simulink model "Main"  (R2021b)
settings: Solver=VariableStepAuto  StartTime=0.0  StopTime=30  MaxStep=0.001  RelTol=1e-3
undefined symbols (not defined in the file): A, B, C, D, F, g, Ixx, Iyy, Izz, ka_lqr, ka_pp, kd_lqr, kd_pp, ks_lqr, ks_pp, L, Lf, m, Q1, Q2, T, u_EP, x_EP, y_EP
libraries: sim3dlib x1, uavsim3dlib x1, matrix_library x1, simulink x1
settings Model: Creator=sina.fazel  LastModifiedBy=Sepiamw

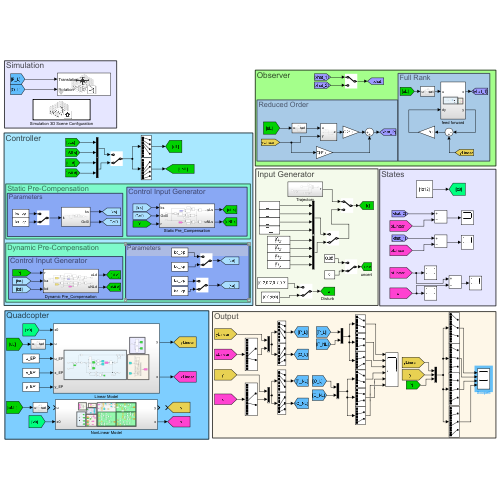
[thumbnail: Simulink's stored preview of the top-level diagram]
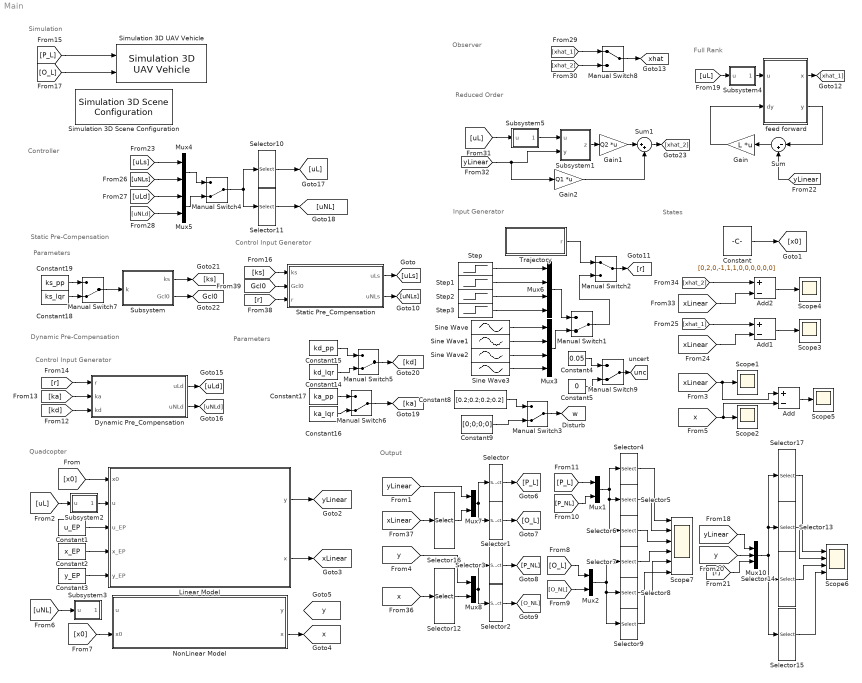
== system Main ==
  note: Full Rank
  note: Observer
  note: Simulation
  note: Control Input Generator
  note: Static Pre-Compensation
  note: Parameters
  note: Controller
  note: States
  note: Output
  note: Quadcopter
  note: Input Generator
  note: Control Input Generator
  note: Dynamic Pre-Compensation
  note: Parameters
  note: Reduced Order
  Add : Sum  Inputs=+-
  Add1 : Sum  Inputs=+-
  Add2 : Sum  Inputs=+-
  Constant : Constant  Value=[0,2,0,-1,1,1,0,0,0,0,0,0]
  Constant1 : Constant  Value=u_EP
  Constant14 : Constant  Value=kd_lqr  VectorParams1D=off
  Constant15 : Constant  Value=kd_pp  VectorParams1D=off
  Constant16 : Constant  Value=ka_lqr  VectorParams1D=off
  Constant17 : Constant  Value=ka_pp  VectorParams1D=off
  Constant18 : Constant  Value=ks_lqr
  Constant19 : Constant  Value=ks_pp
  Constant2 : Constant  Value=x_EP
  Constant3 : Constant  Value=y_EP
  Constant4 : Constant  Value=0.05
  Constant5 : Constant  Value=0
  Constant8 : Constant  Value=[0.2;0.2;0.2;0.2]
  Constant9 : Constant  Value=[0;0;0;0]
  Dynamic Pre_Compensation : Subsystem
  Gain : Gain  Gain=L  Multiplication=Matrix(K*u)
  Gain1 : Gain  Gain=Q2  Multiplication=Matrix(K*u)
  Gain2 : Gain  Gain=Q1  Multiplication=Matrix(K*u)
  Linear Model : Subsystem
  Manual Switch{1,3..7,9} (7 alike) : ManualSwitch  CurrentSetting=0
  Manual Switch2 : ManualSwitch
  Manual Switch8 : ManualSwitch
  Mux{1..2,4..5,7..8} (6 alike) : Mux  Inputs=2
  Mux10 : Mux  Inputs=3
  Mux3 : Mux
  Mux6 : Mux
  NonLinear Model : Subsystem
  Scope{1..5} (5 alike) : Scope
  Scope6 : Scope  NumInputPorts=4
  Scope7 : Scope  NumInputPorts=6
  Selector : Selector  InputPortWidth=6  IndexOptions=Index vector (dialog)  Indices=[1 2 3]  OutputSizes=1
  Selector1 : Selector  InputPortWidth=6  IndexOptions=Index vector (dialog)  Indices=[4 5 6]  OutputSizes=1
  Selector10 : Selector  InputPortWidth=8  IndexOptions=Index vector (dialog)  Indices=[1:4]  OutputSizes=1
  Selector11 : Selector  InputPortWidth=8  IndexOptions=Index vector (dialog)  Indices=[5:8]  OutputSizes=1
  Selector12 : Selector  InputPortWidth=12  IndexOptions=Index vector (dialog)  Indices=[7 8]  OutputSizes=1
  Selector13 : Selector  InputPortWidth=12  IndexOptions=Index vector (dialog)  Indices=[2,6,10]  OutputSizes=1
  Selector14 : Selector  InputPortWidth=12  IndexOptions=Index vector (dialog)  Indices=[3,7,11]  OutputSizes=1
  Selector15 : Selector  InputPortWidth=12  IndexOptions=Index vector (dialog)  Indices=[4,8,12]  OutputSizes=1
  Selector16 : Selector  InputPortWidth=12  IndexOptions=Index vector (dialog)  Indices=[7 8]  OutputSizes=1
  Selector17 : Selector  InputPortWidth=12  IndexOptions=Index vector (dialog)  Indices=[1,5,9]  OutputSizes=1
  Selector2 : Selector  InputPortWidth=6  IndexOptions=Index vector (dialog)  Indices=[4 5 6]  OutputSizes=1
  Selector3 : Selector  InputPortWidth=6  IndexOptions=Index vector (dialog)  Indices=[1 2 3]  OutputSizes=1
  Selector4 : Selector  InputPortWidth=6  IndexOptions=Index vector (dialog)  Indices=[1 4]  OutputSizes=1
  Selector5 : Selector  InputPortWidth=6  IndexOptions=Index vector (dialog)  Indices=[2 5]  OutputSizes=1
  Selector6 : Selector  InputPortWidth=6  IndexOptions=Index vector (dialog)  Indices=[3 6]  OutputSizes=1
  Selector7 : Selector  InputPortWidth=6  IndexOptions=Index vector (dialog)  Indices=[1 4]  OutputSizes=1
  Selector8 : Selector  InputPortWidth=6  IndexOptions=Index vector (dialog)  Indices=[2 5]  OutputSizes=1
  Selector9 : Selector  InputPortWidth=6  IndexOptions=Index vector (dialog)  Indices=[3 6]  OutputSizes=1
  Simulation 3D Scene Configuration : sim3dlib/Simulation 3D Scene Configuration  Priority=0  ProjectFormat_internal=Default Scenes  ProjectFormat=Default Scenes  SceneDesc=US city block  ProjectName=Q:\Matlab\toolbox\shared\sim3d_projects\automotive_project\UE4\WindowsNoEditor\VehicleSimulation.exe  ScenePath=/Game/Maps/USCityBlock  vehTagList={'Drone';'Scene Origin'}  vehTag=Drone  OpVisEn=off  Ts=1/60  EnableWindow=on  EnableWeather=off  SunAltitude=40.0  SunAzimuth=90  clouds=10  wind=1  fog=0  rain=0  sensorTag=MainCamera1  sensorId=1  sensorName=MainCamera1  mountLoc=Origin  offsetFlag=off  tmountOffset=[0, 0, 0]  rmountOffset=[0, 0, 0]  HorizontalResolution=1280  VerticalResolution=720  HorizontalFOV=60  mountPoint=[0 0 0]  mountOrientation=[0 0 0]  aMode=4  ID=1
      settings: SourceProductBaseCode=AE,DR,UV,VE
  Simulation 3D UAV Vehicle : uavsim3dlib/Simulation 3D UAV Vehicle  Priority=-1  Mesh=Quadrotor  MeshPath=/MathWorksUAVContent/UAVs/HexaRotorUAV/HexaRotor.HexaRotor  Color=Black  ActorName=Drone  InitialTranslation=[0 0 1]  InitialRotation=[0 0 0]  SampleTime=-1  ActorType=SimulinkVehicle  ID=C  aMode=4  ActorTag=Drone
      settings: SourceProductBaseCode=UV
  Sine Wave : Sin  Amplitude=0.5  Frequency=pi/8  Phase=pi/4  SampleTime=0
  Sine Wave1 : Sin  Amplitude=0.4  Frequency=pi/8  Phase=pi/8  SampleTime=0
  Sine Wave2 : Sin  Amplitude=1.5  Frequency=pi/8  SampleTime=0
  Sine Wave3 : Sin  Amplitude=0.02  Frequency=pi/16  Phase=pi/8  SampleTime=0
  Static Pre_Compensation : Subsystem
  Step : Step  Time=0  SampleTime=0
  Step1 : Step  Time=0  After=3  SampleTime=0
  Step2 : Step  Time=0  After=4  SampleTime=0
  Step3 : Step  Time=0  After=-pi/32  SampleTime=0
  Subsystem : Subsystem
  Subsystem1 : Subsystem
  Subsystem2 : Subsystem
  Subsystem3 : Subsystem
  Subsystem4 : Subsystem
  Subsystem5 : Subsystem
  Sum : Sum  Inputs=|-+
  Sum1 : Sum  Inputs=|++
  Trajectory : Subsystem
  feed forward : Subsystem
  tag scope: Gcl0=global, unc=global, w=global, x=global, xLinear=global, xhat=global, y=global, yLinear=global
  wires:
  Constant/1 -> [x0]
  Constant3/1 -> Linear Model/5(y_EP)
  Constant2/1 -> Linear Model/4(x_EP)
  Constant1/1 -> Linear Model/3(u_EP)
  Linear Model/1(y) -> [yLinear]
  Linear Model/2(x) -> [xLinear]
  [x0] -> Linear Model/1(x0)
  [xLinear] -> Add/1, Scope1/1
  [x] -> Add/2, Scope2/1
  Selector/1 -> [P_L]
  Selector1/1 -> [O_L]
  Selector3/1 -> [P_NL]
  Selector2/1 -> [O_NL]
  [P_NL] -> Mux1/2
  Add/1 -> Scope5/1
  [P_L] -> Mux1/1
  Mux1/1 -> Selector6/1, Selector5/1, Selector4/1
  Selector6/1 -> Scope7/3
  Selector5/1 -> Scope7/2
  Selector4/1 -> Scope7/1
  [O_L] -> Mux2/1
  [O_NL] -> Mux2/2
  Mux2/1 -> Selector7/1, Selector9/1, Selector8/1
  Selector7/1 -> Scope7/4
  Selector8/1 -> Scope7/5
  Selector9/1 -> Scope7/6
  Manual Switch1/1 -> Manual Switch2/2
  Mux3/1 -> Manual Switch1/2
  Sine Wave/1 -> Mux3/1
  Sine Wave1/1 -> Mux3/2
  Sine Wave2/1 -> Mux3/3
  [uNLs] -> Mux4/2
  [uLs] -> Mux4/1
  [uLd] -> Mux5/1
  [uNLd] -> Mux5/2
  Mux4/1 -> Manual Switch4/1
  Mux5/1 -> Manual Switch4/2
  Selector11/1 -> [uNL]
  Selector10/1 -> [uL]
  Manual Switch4/1 -> Selector10/1, Selector11/1
  Step3/1 -> Mux6/4
  Step2/1 -> Mux6/3
  Step1/1 -> Mux6/2
  Step/1 -> Mux6/1
  Mux6/1 -> Manual Switch1/1
  [y] -> Mux10/2
  [yLinear] -> Mux10/1
  Selector13/1 -> Scope6/2
  Selector15/1 -> Scope6/4
  Selector14/1 -> Scope6/3
  Mux10/1 -> Selector15/1, Selector14/1, Selector17/1, Selector13/1
  Constant8/1 -> Manual Switch3/1
  Constant9/1 -> Manual Switch3/2
  Manual Switch3/1 -> [w]
  Constant14/1 -> Manual Switch5/2
  Constant15/1 -> Manual Switch5/1
  Manual Switch5/1 -> [kd]
  Manual Switch6/1 -> [ka]
  Constant17/1 -> Manual Switch6/1
  Constant16/1 -> Manual Switch6/2
  Sine Wave3/1 -> Mux3/4
  Mux7/1 -> Selector1/1, Selector/1
  Mux8/1 -> Selector3/1, Selector2/1
  [y] -> Mux8/1
  [yLinear] -> Mux7/1
  [x] -> Selector12/1
  Selector12/1 -> Mux8/2
  [xLinear] -> Selector16/1
  Selector16/1 -> Mux7/2
  [r] -> Mux10/3
  Selector17/1 -> Scope6/1
  Constant18/1 -> Manual Switch7/2
  Constant19/1 -> Manual Switch7/1
  Manual Switch7/1 -> Subsystem/1(k)
  Subsystem/1(ks) -> [ks]
  Subsystem/2(Gcl0) -> [Gcl0]
  [ks] -> Static Pre_Compensation/1(ks)
  [r] -> Static Pre_Compensation/3(r)
  [Gcl0] -> Static Pre_Compensation/2(Gcl0)
  Static Pre_Compensation/1(uLs) -> [uLs]
  Static Pre_Compensation/2(uNLs) -> [uNLs]
  Dynamic Pre_Compensation/1(uLd) -> [uLd]
  Dynamic Pre_Compensation/2(uNLd) -> [uNLd]
  [kd] -> Dynamic Pre_Compensation/3(kd)
  [ka] -> Dynamic Pre_Compensation/2(ka)
  [r] -> Dynamic Pre_Compensation/1(r)
  Trajectory/1(r) -> Manual Switch2/1
  Manual Switch2/1 -> [r]
  [P_L] -> Simulation 3D UAV Vehicle/1
  [O_L] -> Simulation 3D UAV Vehicle/2
  NonLinear Model/2(x) -> [x]
  [x0] -> NonLinear Model/2(x0)
  feed forward/1(x) -> [xhat_1]
  feed forward/2(y) -> Sum/1
  [yLinear] -> Sum/2
  Sum/1 -> Gain/1
  Gain/1 -> feed forward/2(dy)
  [xhat_1] -> Add1/1
  [xLinear] -> Add1/2
  Add1/1 -> Scope3/1
  [xhat_1] -> Manual Switch8/1
  [xhat_2] -> Manual Switch8/2
  Manual Switch8/1 -> [xhat]
  [yLinear] -> Gain2/1, Subsystem1/2(y)
  Gain2/1 -> Sum1/2
  Subsystem1/1(z) -> Gain1/1
  Gain1/1 -> Sum1/1
  Sum1/1 -> [xhat_2]
  Add2/1 -> Scope4/1
  [xLinear] -> Add2/2
  [xhat_2] -> Add2/1
  Constant4/1 -> Manual Switch9/1
  Constant5/1 -> Manual Switch9/2
  Manual Switch9/1 -> [unc]
  Subsystem2/1(sat) -> Linear Model/2(u)
  [uL] -> Subsystem2/1(u)
  [uL] -> Subsystem4/1(u)
  Subsystem4/1(sat) -> feed forward/1(u)
  Subsystem5/1(sat) -> Subsystem1/1(u)
  [uL] -> Subsystem5/1(u)
  [uNL] -> Subsystem3/1(u)

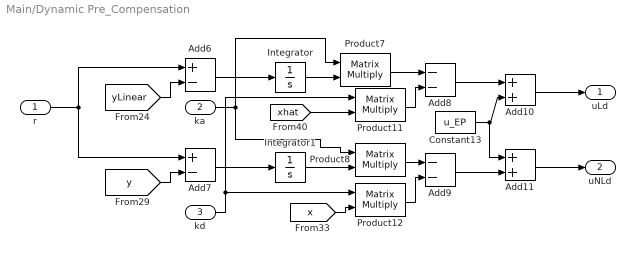
== system Main/Dynamic Pre_Compensation ==
  r : Inport
  ka : Inport  Port=2
  kd : Inport  Port=3
  Add10 : Sum
  Add11 : Sum
  Add6 : Sum  Inputs=+-
  Add7 : Sum  Inputs=+-
  Add8 : Sum  Inputs=--
  Add9 : Sum  Inputs=--
  Constant13 : Constant  Value=u_EP
  Integrator : Integrator
  Integrator1 : Integrator
  Product{7..8,11..12} (4 alike) : Product  Multiplication=Matrix(*)
  uLd : Outport
  uNLd : Outport  Port=2
  wires:
  Product12/1 -> Add9/2
  [xhat] -> Product11/2
  Product11/1 -> Add8/2
  kd/1 -> Product12/1, Product11/1
  ka/1 -> Product8/1, Product7/1
  [x] -> Product12/2
  Integrator/1 -> Product7/2
  Product7/1 -> Add8/1
  Constant13/1 -> Add11/1, Add10/2
  Add11/1 -> uNLd/1
  Add8/1 -> Add10/1
  Add9/1 -> Add11/2
  Integrator1/1 -> Product8/2
  Add10/1 -> uLd/1
  Product8/1 -> Add9/1
  Add7/1 -> Integrator1/1
  [y] -> Add7/2
  r/1 -> Add7/1, Add6/1
  [yLinear] -> Add6/2
  Add6/1 -> Integrator/1

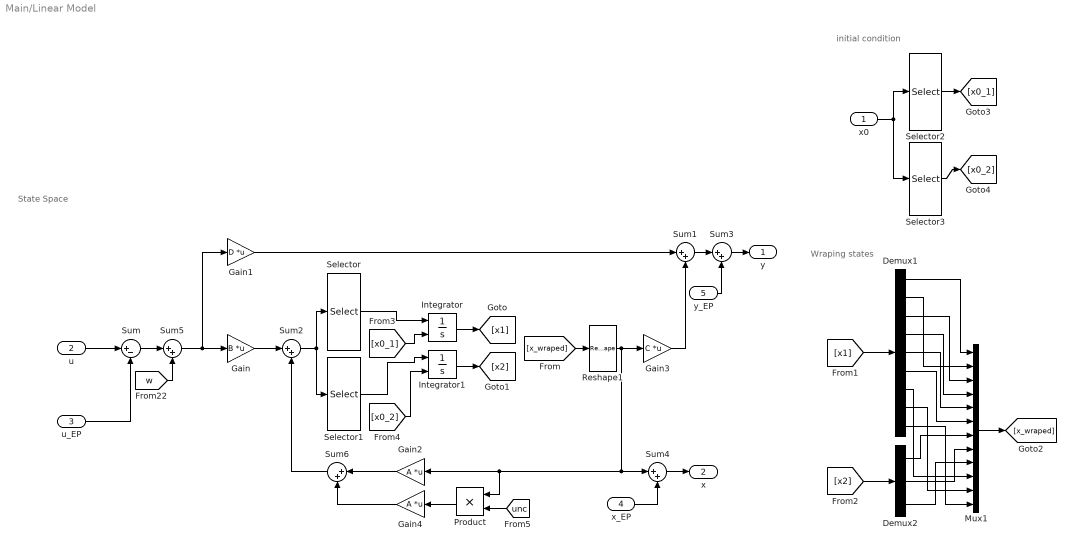
== system Main/Linear Model ==
  note: State Space
  note: Wraping states
  note: initial condition
  x0 : Inport
  u : Inport  Port=2
  u_EP : Inport  Port=3
  x_EP : Inport  Port=4
  y_EP : Inport  Port=5
  Demux1 : Demux  Outputs=9
  Demux2 : Demux  Outputs=3
  Gain : Gain  Gain=B  Multiplication=Matrix(K*u)
  Gain1 : Gain  Gain=D  Multiplication=Matrix(K*u)
  Gain2 : Gain  Gain=A  Multiplication=Matrix(K*u)
  Gain3 : Gain  Gain=C  Multiplication=Matrix(K*u)
  Gain4 : Gain  Gain=A  Multiplication=Matrix(K*u)
  Integrator : Integrator  InitialConditionSource=external
  Integrator1 : Integrator  InitialConditionSource=external  WrapState=on
  Mux1 : Mux  Inputs=12
  Product : Product
  Reshape1 : Reshape  OutputDimensionality=Column vector (2-D)
  Selector : Selector  InputPortWidth=12  IndexOptions=Index vector (dialog)  Indices=[1 2 3 4 5 6 10 11 12]  OutputSizes=1
  Selector1 : Selector  InputPortWidth=12  IndexOptions=Index vector (dialog)  Indices=[7 8 9]  OutputSizes=1
  Selector2 : Selector  InputPortWidth=12  IndexOptions=Index vector (dialog)  Indices=[1 2 3 4 5 6 10 11 12]  OutputSizes=1
  Selector3 : Selector  InputPortWidth=12  IndexOptions=Index vector (dialog)  Indices=[7 8 9]  OutputSizes=1
  Sum : Sum  Inputs=|+-
  Sum{1..6} (6 alike) : Sum  Inputs=|++
  y : Outport
  x : Outport  Port=2
  wires:
  [x1] -> Demux1/1
  Demux1/9 -> Mux1/12
  Demux1/5 -> Mux1/5
  [x2] -> Demux2/1
  Demux1/4 -> Mux1/4
  Demux2/2 -> Mux1/8
  Demux1/1 -> Mux1/1
  Demux1/7 -> Mux1/10
  Demux1/6 -> Mux1/6
  Demux1/3 -> Mux1/3
  Demux1/2 -> Mux1/2
  Demux2/3 -> Mux1/9
  Demux1/8 -> Mux1/11
  Demux2/1 -> Mux1/7
  Mux1/1 -> [x_wraped]
  x0/1 -> Selector3/1, Selector2/1
  Selector2/1 -> [x0_1]
  Selector3/1 -> [x0_2]
  Sum2/1 -> Selector1/1, Selector/1
  Selector/1 -> Integrator/1
  y_EP/1 -> Sum3/2
  Gain1/1 -> Sum1/1
  Sum3/1 -> y/1
  Gain/1 -> Sum2/1
  x_EP/1 -> Sum4/2
  Selector1/1 -> Integrator1/1
  [x0_1] -> Integrator/2
  [x0_2] -> Integrator1/2
  u/1 -> Sum/1
  Integrator/1 -> [x1]
  Sum1/1 -> Sum3/1
  Integrator1/1 -> [x2]
  u_EP/1 -> Sum/2
  Gain3/1 -> Sum1/2
  Sum4/1 -> x/1
  Sum/1 -> Sum5/1
  Sum5/1 -> Gain1/1, Gain/1
  [x_wraped] -> Reshape1/1
  Reshape1/1 -> Sum4/1, Product/1, Gain2/1, Gain3/1
  [w] -> Sum5/2
  Gain2/1 -> Sum6/1
  Sum6/1 -> Sum2/2
  Product/1 -> Gain4/1
  Gain4/1 -> Sum6/2
  [unc] -> Product/2

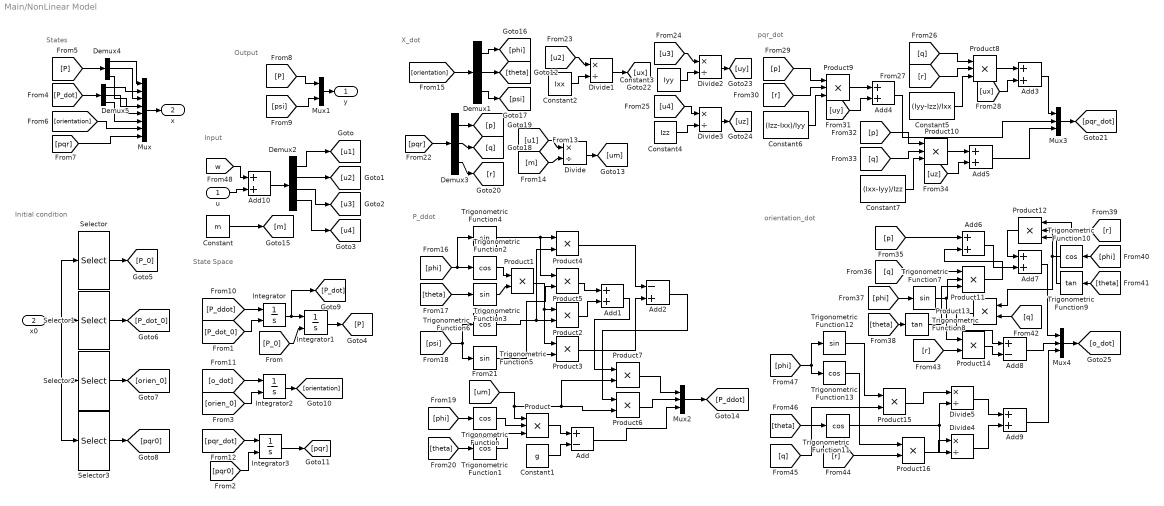
== system Main/NonLinear Model ==
  note: X_dot
  note: P_ddot
  note: State Space
  note: Output
  note: States
  note: Input
  note: Initial condition
  note: pqr_dot
  note: orientation_dot
  u : Inport
  x0 : Inport  Port=2
  Add : Sum  Inputs=+-
  Add{1,3..7,9..10} (8 alike) : Sum
  Add2 : Sum  Inputs=-+
  Add8 : Sum  Inputs=+-
  Constant : Constant  Value=m
  Constant1 : Constant  Value=g
  Constant2 : Constant  Value=Ixx
  Constant3 : Constant  Value=Iyy
  Constant4 : Constant  Value=Izz
  Constant5 : Constant  Value=(Iyy-Izz)/Ixx
  Constant6 : Constant  Value=(Izz-Ixx)/Iyy
  Constant7 : Constant  Value=(Ixx-Iyy)/Izz
  Demux{1,3..5} (4 alike) : Demux  Outputs=3
  Demux2 : Demux
  Divide{,1..5} (6 alike) : Product  Inputs=*/
  Integrator : Integrator  InitialConditionSource=external
  Integrator1 : Integrator  InitialConditionSource=external
  Integrator2 : Integrator  InitialConditionSource=external  WrapState=on
  Integrator3 : Integrator  InitialConditionSource=external
  Mux : Mux  Inputs=8
  Mux1 : Mux  Inputs=2
  Mux2 : Mux  Inputs=3
  Mux3 : Mux  Inputs=3
  Mux4 : Mux  Inputs=3
  Product{,8..12} (6 alike) : Product  Inputs=3
  Product{1..7,13..16} (11 alike) : Product
  Selector : Selector  InputPortWidth=12  IndexOptions=Index vector (dialog)  Indices=[1 3 5]  OutputSizes=1
  Selector1 : Selector  InputPortWidth=12  IndexOptions=Index vector (dialog)  Indices=[2 4 6]  OutputSizes=1
  Selector2 : Selector  InputPortWidth=12  IndexOptions=Index vector (dialog)  Indices=[7 8 9]  OutputSizes=1
  Selector3 : Selector  InputPortWidth=12  IndexOptions=Index vector (dialog)  Indices=[10 11 12]  OutputSizes=1
  Trigonometric Function{,1..2,6,10..11,13} (7 alike) : Trigonometry  Operator=cos
  Trigonometric Function{3..5,7,12} (5 alike) : Trigonometry
  Trigonometric Function8 : Trigonometry  Operator=tan
  Trigonometric Function9 : Trigonometry  Operator=tan
  y : Outport
  x : Outport  Port=2
  wires:
  x0/1 -> Selector3/1, Selector2/1, Selector1/1, Selector/1
  u/1 -> Add10/2
  Demux2/1 -> [u1]
  Demux2/4 -> [u4]
  Demux2/3 -> [u3]
  Demux2/2 -> [u2]
  Integrator/1 -> [P_dot], Integrator1/1
  Selector/1 -> [P_0]
  Selector1/1 -> [P_dot_0]
  [P_0] -> Integrator1/2
  [P_dot_0] -> Integrator/2
  Selector2/1 -> [orien_0]
  Selector3/1 -> [pqr0]
  [pqr0] -> Integrator3/2
  [orien_0] -> Integrator2/2
  Integrator1/1 -> [P]
  Integrator2/1 -> [orientation]
  Integrator3/1 -> [pqr]
  [pqr] -> Mux/8
  [orientation] -> Mux/7
  [P_dot] -> Demux5/1
  [P] -> Demux4/1
  Mux/1 -> x/1
  Mux1/1 -> y/1
  [P] -> Mux1/1
  [P_ddot] -> Integrator/1
  [o_dot] -> Integrator2/1
  [pqr_dot] -> Integrator3/1
  Constant/1 -> [m]
  [u1] -> Divide/1
  Demux1/3 -> [psi]
  Demux1/2 -> [theta]
  Demux1/1 -> [phi]
  [m] -> Divide/2
  Divide/1 -> [um]
  [orientation] -> Demux1/1
  [phi] -> Trigonometric Function/1
  [theta] -> Trigonometric Function1/1
  [um] -> Product7/2, Product6/2, Product/1
  Trigonometric Function/1 -> Product/2
  Trigonometric Function1/1 -> Product/3
  Product/1 -> Add/1
  Constant1/1 -> Add/2
  [pqr] -> Demux3/1
  Demux3/2 -> [q]
  Demux3/3 -> [r]
  Demux3/1 -> [p]
  Add/1 -> Mux2/3
  Mux2/1 -> [P_ddot]
  [phi] -> Trigonometric Function4/1, Trigonometric Function2/1
  [theta] -> Trigonometric Function3/1
  Trigonometric Function2/1 -> Product1/1
  Trigonometric Function3/1 -> Product1/2
  [psi] -> Trigonometric Function5/1, Trigonometric Function6/1
  Product1/1 -> Product3/1, Product2/1
  Trigonometric Function6/1 -> Product4/2, Product2/2
  Trigonometric Function5/1 -> Product3/2, Product5/2
  Trigonometric Function4/1 -> Product5/1, Product4/1
  Product2/1 -> Add1/2
  Product5/1 -> Add1/1
  Product3/1 -> Add2/2
  Product4/1 -> Add2/1
  Product7/1 -> Mux2/1
  Product6/1 -> Mux2/2
  Add2/1 -> Product6/1
  Add1/1 -> Product7/1
  Mux3/1 -> [pqr_dot]
  Constant4/1 -> Divide3/2
  Constant3/1 -> Divide2/2
  [u4] -> Divide3/1
  [u3] -> Divide2/1
  [u2] -> Divide1/1
  Constant2/1 -> Divide1/2
  Divide1/1 -> [ux]
  Divide2/1 -> [uy]
  Divide3/1 -> [uz]
  [q] -> Product8/1
  [r] -> Product8/2
  Product8/1 -> Add3/1
  Constant5/1 -> Product8/3
  [ux] -> Add3/2
  Add3/1 -> Mux3/1
  [uy] -> Add4/2
  Constant6/1 -> Product9/3
  Product9/1 -> Add4/1
  [r] -> Product9/2
  [p] -> Product9/1
  Add4/1 -> Mux3/2
  [p] -> Product10/1
  [q] -> Product10/2
  Product10/1 -> Add5/1
  Constant7/1 -> Product10/3
  [uz] -> Add5/2
  Add5/1 -> Mux3/3
  Mux4/1 -> [o_dot]
  [p] -> Add6/1
  [q] -> Product11/1
  Product11/1 -> Add6/2
  Trigonometric Function7/1 -> Product14/1, Product11/2
  [phi] -> Trigonometric Function7/1
  [theta] -> Trigonometric Function8/1
  Trigonometric Function8/1 -> Product11/3
  Add6/1 -> Add7/2
  Add7/1 -> Mux4/1
  [theta] -> Trigonometric Function9/1
  Product12/1 -> Add7/1
  [phi] -> Trigonometric Function10/1
  Trigonometric Function10/1 -> Product13/1, Product12/2
  Trigonometric Function9/1 -> Product12/3
  [r] -> Product12/1
  [q] -> Product13/2
  Add8/1 -> Mux4/2
  Product13/1 -> Add8/1
  Product14/1 -> Add8/2
  [r] -> Product14/2
  Add9/1 -> Mux4/3
  [r] -> Product16/2
  [q] -> Product15/2
  [theta] -> Trigonometric Function11/1
  Trigonometric Function11/1 -> Divide4/2, Divide5/2
  Product16/1 -> Divide4/1
  Product15/1 -> Divide5/1
  Divide5/1 -> Add9/1
  Divide4/1 -> Add9/2
  [phi] -> Trigonometric Function12/1, Trigonometric Function13/1
  Trigonometric Function12/1 -> Product15/1
  Trigonometric Function13/1 -> Product16/1
  Demux5/3 -> Mux/6
  Demux5/2 -> Mux/4
  Demux5/1 -> Mux/2
  Demux4/1 -> Mux/1
  Demux4/2 -> Mux/3
  Demux4/3 -> Mux/5
  Add10/1 -> Demux2/1
  [w] -> Add10/1
  [psi] -> Mux1/2

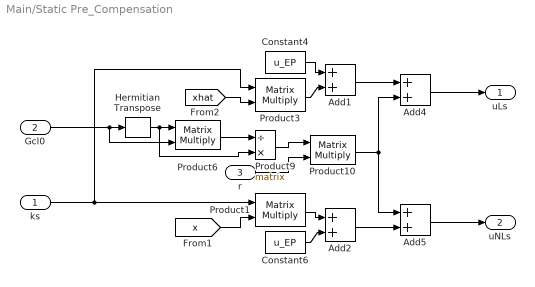
== system Main/Static Pre_Compensation ==
  ks : Inport
  Gcl0 : Inport  Port=2
  r : Inport  Port=3
  Add{1..2,4..5} (4 alike) : Sum
  Constant4 : Constant  Value=u_EP
  Constant6 : Constant  Value=u_EP
  Hermitian Transpose : matrix_library/Hermitian Transpose
      settings: SourceProductBaseCode=SL
  Product{1,3,6,10} (4 alike) : Product  Multiplication=Matrix(*)
  Product9 : Product  Inputs=/*  Multiplication=Matrix(*)
  uLs : Outport
  uNLs : Outport  Port=2
  wires:
  Gcl0/1 -> Product6/2, Hermitian Transpose/1
  Product6/1 -> Product9/1
  [xhat] -> Product3/2
  ks/1 -> Product1/1, Product3/1
  Product1/1 -> Add2/1
  Product9/1 -> Product10/1
  Constant4/1 -> Add1/1
  r/1 -> Product10/2
  [x] -> Product1/2
  Hermitian Transpose/1 -> Product9/2, Product6/1
  Add2/1 -> Add5/2
  Add1/1 -> Add4/1
  Add5/1 -> uNLs/1
  Product10/1 -> Add4/2, Add5/1
  Product3/1 -> Add1/2
  Add4/1 -> uLs/1
  Constant6/1 -> Add2/2

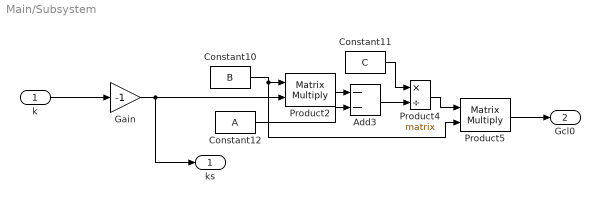
== system Main/Subsystem ==
  k : Inport
  Add3 : Sum  Inputs=--
  Constant10 : Constant  Value=B  VectorParams1D=off
  Constant11 : Constant  Value=C  VectorParams1D=off
  Constant12 : Constant  Value=A  VectorParams1D=off
  Gain : Gain  Gain=-1
  Product2 : Product  Multiplication=Matrix(*)
  Product4 : Product  Inputs=*/  Multiplication=Matrix(*)
  Product5 : Product  Multiplication=Matrix(*)
  ks : Outport
  Gcl0 : Outport  Port=2
  wires:
  Constant10/1 -> Product2/1, Product5/2
  Add3/1 -> Product4/2
  Gain/1 -> ks/1, Product2/2
  Constant11/1 -> Product4/1
  Product2/1 -> Add3/1
  Constant12/1 -> Add3/2
  Product5/1 -> Gcl0/1
  Product4/1 -> Product5/1
  k/1 -> Gain/1

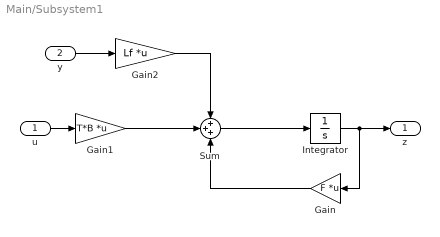
== system Main/Subsystem1 ==
  u : Inport
  y : Inport  Port=2
  Gain : Gain  Gain=F  Multiplication=Matrix(K*u)
  Gain1 : Gain  Gain=T*B  Multiplication=Matrix(K*u)
  Gain2 : Gain  Gain=Lf  Multiplication=Matrix(K*u)
  Integrator : Integrator
  Sum : Sum  Inputs=+++
  z : Outport
  wires:
  Integrator/1 -> Gain/1, z/1
  Sum/1 -> Integrator/1
  Gain/1 -> Sum/3
  Gain1/1 -> Sum/2
  u/1 -> Gain1/1
  y/1 -> Gain2/1
  Gain2/1 -> Sum/1

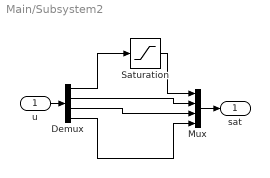
== system Main/Subsystem2 ==
  u : Inport
  Demux : Demux
  Mux : Mux
  Saturation : Saturate  UpperLimit=35  LowerLimit=0
  sat : Outport
  wires:
  Demux/4 -> Mux/4
  Demux/3 -> Mux/3
  Demux/2 -> Mux/2
  Saturation/1 -> Mux/1
  Demux/1 -> Saturation/1
  u/1 -> Demux/1
  Mux/1 -> sat/1

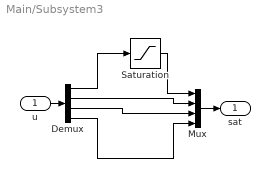
== system Main/Subsystem3 ==
  u : Inport
  Demux : Demux
  Mux : Mux
  Saturation : Saturate  UpperLimit=25  LowerLimit=0
  sat : Outport
  wires:
  Demux/4 -> Mux/4
  Demux/3 -> Mux/3
  Demux/2 -> Mux/2
  Saturation/1 -> Mux/1
  Demux/1 -> Saturation/1
  u/1 -> Demux/1
  Mux/1 -> sat/1

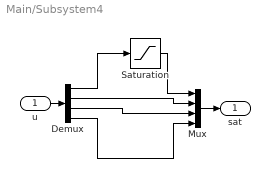
== system Main/Subsystem4 ==
  u : Inport
  Demux : Demux
  Mux : Mux
  Saturation : Saturate  UpperLimit=35  LowerLimit=0
  sat : Outport
  wires:
  Demux/4 -> Mux/4
  Demux/3 -> Mux/3
  Demux/2 -> Mux/2
  Saturation/1 -> Mux/1
  Demux/1 -> Saturation/1
  u/1 -> Demux/1
  Mux/1 -> sat/1

== system Main/Subsystem5 ==
  u : Inport
  Demux : Demux
  Mux : Mux
  Saturation : Saturate  UpperLimit=25  LowerLimit=0
  sat : Outport
  wires:
  Demux/4 -> Mux/4
  Demux/3 -> Mux/3
  Demux/2 -> Mux/2
  Saturation/1 -> Mux/1
  Demux/1 -> Saturation/1
  u/1 -> Demux/1
  Mux/1 -> sat/1

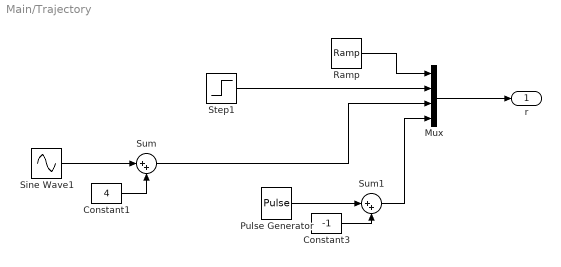
== system Main/Trajectory ==
  Constant1 : Constant  Value=4
  Constant3 : Constant  Value=-1
  Mux : Mux
  Pulse Generator : DiscretePulseGenerator  PulseType=Time based  Amplitude=2  Period=8  PulseWidth=50
  Ramp : simulink/Sources/Ramp  slope=4  start=0  InitialOutput=0
  Sine Wave1 : Sin  Amplitude=2  Frequency=pi/4  SampleTime=0
  Step1 : Step  Time=4  SampleTime=0
  Sum : Sum  Inputs=|++
  Sum1 : Sum  Inputs=|++
  r : Outport
  wires:
  Mux/1 -> r/1
  Sum1/1 -> Mux/4
  Sine Wave1/1 -> Sum/1
  Constant1/1 -> Sum/2
  Constant3/1 -> Sum1/2
  Pulse Generator/1 -> Sum1/1
  Sum/1 -> Mux/3
  Step1/1 -> Mux/2
  Ramp/1 -> Mux/1

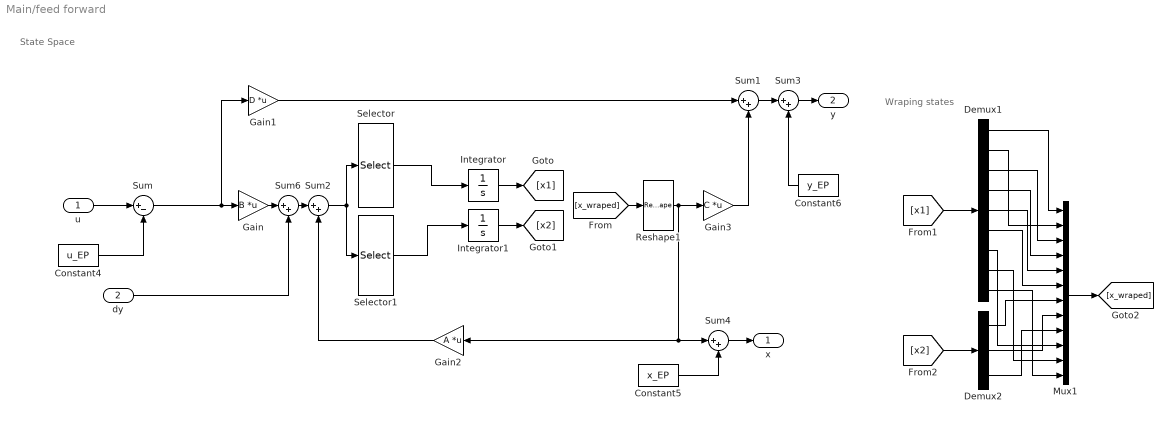
== system Main/feed forward ==
  note: Wraping states
  note: State Space
  u : Inport
  dy : Inport  Port=2
  Constant4 : Constant  Value=u_EP
  Constant5 : Constant  Value=x_EP
  Constant6 : Constant  Value=y_EP
  Demux1 : Demux  Outputs=9
  Demux2 : Demux  Outputs=3
  Gain : Gain  Gain=B  Multiplication=Matrix(K*u)
  Gain1 : Gain  Gain=D  Multiplication=Matrix(K*u)
  Gain2 : Gain  Gain=A  Multiplication=Matrix(K*u)
  Gain3 : Gain  Gain=C  Multiplication=Matrix(K*u)
  Integrator : Integrator
  Integrator1 : Integrator  WrapState=on
  Mux1 : Mux  Inputs=12
  Reshape1 : Reshape  OutputDimensionality=Column vector (2-D)
  Selector : Selector  InputPortWidth=12  IndexOptions=Index vector (dialog)  Indices=[1 2 3 4 5 6 10 11 12]  OutputSizes=1
  Selector1 : Selector  InputPortWidth=12  IndexOptions=Index vector (dialog)  Indices=[7 8 9]  OutputSizes=1
  Sum : Sum  Inputs=|+-
  Sum{1..4,6} (5 alike) : Sum  Inputs=|++
  x : Outport
  y : Outport  Port=2
  wires:
  Reshape1/1 -> Gain3/1, Gain2/1, Sum4/1
  [x_wraped] -> Reshape1/1
  Sum/1 -> Gain/1, Gain1/1
  Gain2/1 -> Sum2/2
  Sum4/1 -> x/1
  Gain3/1 -> Sum1/2
  Integrator1/1 -> [x2]
  Sum1/1 -> Sum3/1
  Integrator/1 -> [x1]
  u/1 -> Sum/1
  Selector1/1 -> Integrator1/1
  Gain/1 -> Sum6/1
  Sum3/1 -> y/1
  Gain1/1 -> Sum1/1
  Selector/1 -> Integrator/1
  Sum2/1 -> Selector/1, Selector1/1
  Mux1/1 -> [x_wraped]
  Demux2/1 -> Mux1/7
  Demux1/8 -> Mux1/11
  Demux2/3 -> Mux1/9
  Demux1/2 -> Mux1/2
  Demux1/3 -> Mux1/3
  Demux1/6 -> Mux1/6
  Demux1/7 -> Mux1/10
  Demux1/1 -> Mux1/1
  Demux2/2 -> Mux1/8
  Demux1/4 -> Mux1/4
  [x2] -> Demux2/1
  Demux1/5 -> Mux1/5
  Demux1/9 -> Mux1/12
  [x1] -> Demux1/1
  Constant4/1 -> Sum/2
  Constant5/1 -> Sum4/2
  Constant6/1 -> Sum3/2
  dy/1 -> Sum6/2
  Sum6/1 -> Sum2/1
